simulink model "PowerLimiting_Saturation_LowPower"  (R2024a)
settings: Solver=VariableStepAuto  StartTime=0.0  StopTime=10  RelTol=1e-3
undefined symbols (not defined in the file or in its folder): Ion, Lithium
libraries: spsBatteryLib x1, spsControlledCurrentSourceLib x1, slpidlib x1, dspstat3 x1, spsVoltageMeasurementLib x1, simulink x1, sps_lib x1
settings Model: Creator=ezeki  LastModifiedBy=ezeki
settings DataIOCC: ExternalInput=[throttle]

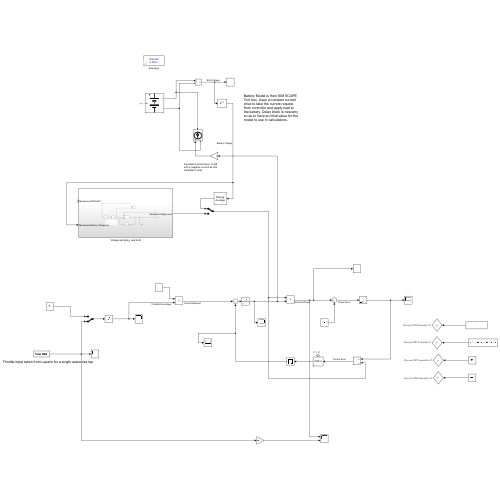
[thumbnail: Simulink's stored preview of the top-level diagram]
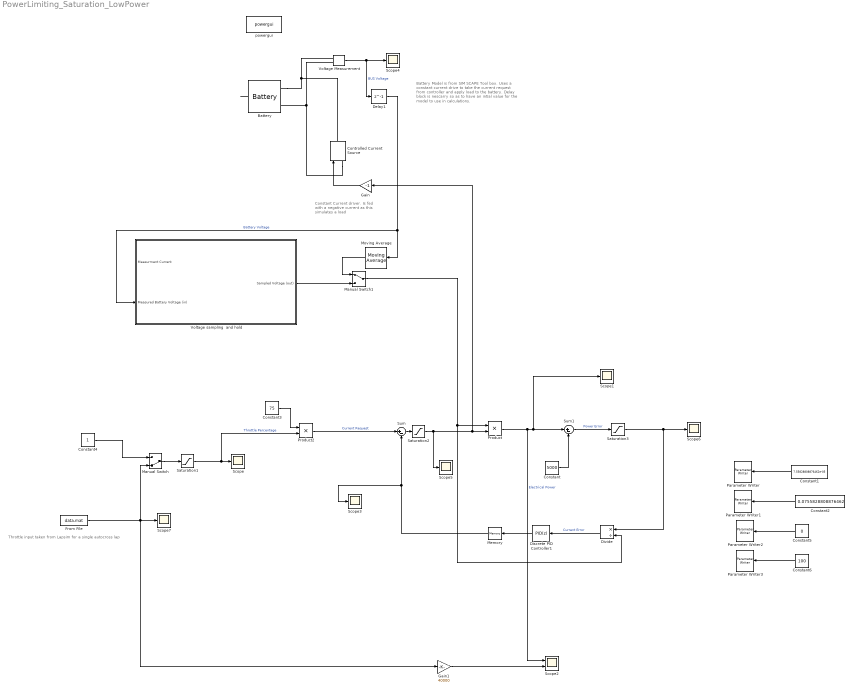
== system PowerLimiting_Saturation_LowPower ==
  note: Throttle input taken from Lapsim for a single autocross lap
  note: Constant Current driver. Is fed with a negative current as this simulates a load
  note: Battery Model is from SIM SCAPE Tool box. Uses a constant current drive to take the current request from controller and apply load to the battery. Delay block is nescarry so as to have an intial value for the model to use in calculations.
  Battery : spsBatteryLib/Battery  BatType=Lithium-Ion  ShowTempParam=off  ThermalPreset=no  ShowAgeParam=off  NomV=532.8  NomQ=1152  SOC=98.5  Batt_Tr=5  PresetModel=on  MaxQ=1152  MinV=399.6  FullV=620.1723  Dis_rate=500.8696  R=0.004625  Normal_OP=1041.8087  expZone="[575.6296      56.59826]"  current=[6.5 13 32.5]  Units=Time  Tci=20  NomT=20  T2=-30  MaxQ2=4.8  FullV2=7.1  Normal_OP2=5.655  expZone2="[6.58           1]"  Rca=0.6  ti=2000  Dp=0  Neq0=0  Tsim=1e6  Ta1=25  Qeol=5.4*0.9  Reol=0.013333*1.2  Char_age=[2.3478, 3]  Dis_age=[2.3478, 10]  N1=1500  N2=10500  N3=1000  N4=1400  Ta2=45  N5=950
  Constant : Constant  Value=5000
  Constant1 : Constant  Value=7.55828808876462e-05
  Constant2 : Constant  Value=0.0755828808876462
  Constant3 : Constant  Value=75
  Constant4 : Constant
  Constant5 : Constant  Value=0
  Constant6 : Constant  Value=100
  Controlled Current Source : spsControlledCurrentSourceLib/Controlled Current Source  Initialize=on  Source_Type=AC  Amplitude=0  Phase=0  Frequency=0  Measurements=None
  Delay1 : Delay  DelayLength=1  InitialCondition=600
  Discrete PID Controller1 : slpidlib/PID Controller  Controller=PID  Form=Parallel  TimeDomain=Discrete-time  UseExternalTs=off  SampleTime=-1  IntegratorMethod=Forward Euler  FilterMethod=Forward Euler  ControllerParametersSource=internal  P=1  I=1  UseKiTs=on  D=0  UseExternalDerivativeSource=off  N=100  UseFilter=on  TunerSelectOption=Transfer Function Based (PID Tuner App)  InitialConditionSource=internal  InitialConditionForIntegrator=60  InitialConditionForFilter=0  DifferentiatorICPrevScaledInput=0  ExternalReset=none  TrackingMode=off  Kt=1  LimitOutput=off  SatLimitsSource=internal  UpperSaturationLimit=inf  LowerSaturationLimit=-inf  LinearizeAsGain=off  AntiWindupMode=none  Kb=1  LimitIntegrator=off  UpperIntegratorSaturationLimit=inf  LowerIntegratorSaturationLimit=-inf  POutMin=[]  POutMax=[]  IOutMin=[]  IOutMax=[]  DOutMin=[]  DOutMax=[]  NOutMin=[]  NOutMax=[]  SumOutMin=[]  SumOutMax=[]  SaturationOutMin=[]  SaturationOutMax=[]  PParamMin=[]  PParamMax=[]  IParamMin=[]  IParamMax=[]  DParamMin=[]  DParamMax=[]  NParamMin=[]  NParamMax=[]  KbParamMin=[]  KbParamMax=[]  KtParamMin=[]  KtParamMax=[]  KbOutMin=[]  KbOutMax=[]  KtOutMin=[]  KtOutMax=[]  IntegratorOutMin=[]  IntegratorOutMax=[]  FilterOutMin=[]  FilterOutMax=[]  SumI1OutMin=[]  SumI1OutMax=[]  SumI2OutMin=[]  SumI2OutMax=[]  SumI3OutMin=[]  SumI3OutMax=[]  SumI4OutMin=[]  SumI4OutMax=[]  SumDOutMin=[]  SumDOutMax=[]  DifferentiatorOutMin=[]  DifferentiatorOutMax=[]  FilterDiffOutCoefMin=[]  FilterDiffOutCoefMax=[]  ReciprocalOutMin=[]  ReciprocalOutMax=[]  SumDenOutMin=[]  SumDenOutMax=[]  SumNumOutMin=[]  SumNumOutMax=[]  DivideOutMin=[]  DivideOutMax=[]  UdiffTsProdOutMin=[]  UdiffTsProdOutMax=[]  NTsProdOutMin=[]  NTsProdOutMax=[]  UintegralTsProdOutMin=[]  UintegralTsProdOutMax=[]  UngainTsProdOutMin=[]  UngainTsProdOutMax=[]  ClampingZeroOutDataTypeStr=Inherit: Inherit via back propagation  ClampingZeroOutMin=[]  ClampingZeroOutMax=[]  FilterDenConstantOutDataTypeStr=Inherit: Inherit via back propagation  FilterDenConstantOutMin=[]  FilterDenConstantOutMax=[]  PCopyOutDataTypeStr=Inherit: Inherit via back propagation  PCopyOutMin=[]  PCopyOutMax=[]  NCopyOutDataTypeStr=Inherit: Inherit via back propagation  NCopyOutMin=[]  NCopyOutMax=[]  IntegratorContinuousStateAttributes=''  IntegratorStateMustResolveToSignalObject=off  IntegratorRTWStateStorageClass=Auto  FilterContinuousStateAttributes=''  FilterStateMustResolveToSignalObject=off  FilterRTWStateStorageClass=Auto  ParallelPVariant=InternalParameters  IdealPVariant=Disabled  IVariant=InternalParameters  DVariant=InternalParameters  IntegratorVariant=Discrete  SatVariant=Disabled  AWVariant=Passthrough  PCopyVariant=Disabled  TRVariant=Disabled  FdbkBlocksVariant=Forward  IdealPFdbkVariant=Disabled  SatFdbkVariant=Disabled  DerivativeFilterVariant=ForwardEulerFilter  NVariant=InternalParameters  NCopyVariant=Disabled  FilterICVariant=InternalICsFilter  IntegratorICVariant=InternalICs  ExternalResetVariant=Disabled  TRSumVariant=Passthrough  SumFdbkVariant=Disabled  SumVariant=Sum_PID  TsampFilterVariant=InternalTs  TsampNgainVariant=Passthrough  TsampIntegralVariant=Disabled_SignalSpec  ExternalSaturationOutDataTypeStr=Inherit: Same as second input  DerivativeSourceVariant=ErrorSignal
      settings: LibrarySourceBlock=simulink/Discrete/Discrete PID Controller
  Divide : Product  Inputs=*/
  From File : FromFile  FileName=data.mat  SampleTime=0
  Gain : Gain  Gain=-1
  Gain1 : Gain  Gain=40000
  Manual Switch : ManualSwitch  CurrentSetting=0
  Manual Switch1 : ManualSwitch
  Memory : Memory  InitialCondition=14
  Moving Average : dspstat3/Moving Average  Method=Sliding window  ForgettingFactorPort=off  SpecifyWindowLength=on  WindowLength=10  OverlapLength=9  AllowArbitraryInputLength=off  ForgettingFactor=0.9  SimulateUsing=Interpreted execution
  Parameter Writer : ParameterWriter  ParameterOwnerBlock=../Discrete PID Controller1  ParameterName=P  ParameterInternalName=P
  Parameter Writer1 : ParameterWriter  ParameterOwnerBlock=../Discrete PID Controller1  ParameterName=I  ParameterInternalName=I
  Parameter Writer2 : ParameterWriter  ParameterOwnerBlock=../Discrete PID Controller1  ParameterName=D  ParameterInternalName=D
  Parameter Writer3 : ParameterWriter  ParameterOwnerBlock=../Discrete PID Controller1  ParameterName=N  ParameterInternalName=N
  Product : Product
  Product2 : Product
  Saturation1 : Saturate  UpperLimit=inf  LowerLimit=0
  Saturation2 : Saturate  UpperLimit=inf  LowerLimit=0
  Saturation3 : Saturate  UpperLimit=inf  LowerLimit=0
  Scope{,1,3..7} (7 alike) : Scope
  Scope2 : Scope  NumInputPorts=2
  Sum : Sum  Inputs=|+-
  Sum1 : Sum  Inputs=|+-
  Voltage Measurement : spsVoltageMeasurementLib/Voltage Measurement  PhasorSimulation=off  OutputType=Complex  PSBequivalent=0
  Voltage sampling  and hold : Subsystem
  powergui : sps_lib/powergui  Priority=1  SimulationMode=Discrete  SampleTime=0.002  frequency=60  Iterations=50  frequencyindice=0  Pbase=100e6  ErrMax=1e-4  UnitsV=kV  UnitsW=MW  buscounter=0  FunctionMessages=off  echomessages=off  EnableUseOfTLC=off  CurrentSourceSwitches=off  DisableSnubberDevices=off  DisableRonSwitches=off  DisableVfSwitches=off  DisplayEquations=off  AutomaticDiscreteSolvers=off  SolverType=Tustin/Backward Euler (TBE)  Interpol=off  ExternalGateDelay=off  methode=off  Ts=100  x0status=blocks  SPID=on  SwTol=0  HookPort=off  NonlinearTolerance=1e-4  nMaxIteration=100  ContinueOnMaxIteration=off  RestoreLinks=warning  ResistiveCurrentMeasurement=off  Frange=[0:2:500]  Ylog=off  Xlog=on  ShowGrid=off  save=off  variable=ZData  structure=0  ZoomFFT=off  StartTime=0.0  cycles=1  DisplayStyle=1  fundamental=60  FreqAxis=off  MaxFrequency=1000  frequencyindicesteady=1  RmsSteady=1  display=off
  wires:
  Saturation1/1 -> Scope/1, Product2/2  "Throttle Percentage"
  Constant4/1 -> Manual Switch/1
  Manual Switch/1 -> Saturation1/1
  Constant3/1 -> Product2/1
  Gain/1 -> Controlled Current Source/1
  Voltage Measurement/1 -> Delay1/1, Scope4/1  "BUS Voltage"
  Delay1/1 -> Voltage sampling  and hold/2(Measured Battery Voltage (in)), Moving Average/1  "Battery Voltage"
  Battery/1 -> ?
  From File/1 -> Manual Switch/2, Gain1/1, Scope7/1
  Product2/1 -> Sum/1  "Current Request"
  Voltage sampling  and hold/1(Sampled Voltage (out)) -> Manual Switch1/2
  Manual Switch1/1 -> Divide/2, Product/1
  Product/1 -> Scope1/1, Sum1/1, Scope2/1  "Electrical Power"
  Constant/1 -> Sum1/2
  Sum1/1 -> Saturation3/1  "Power Error"
  Divide/1 -> Discrete PID Controller1/1  "Current Error"
  Discrete PID Controller1/1 -> Memory/1
  Saturation2/1 -> Scope5/1, Gain/1, Product/2
  Moving Average/1 -> Manual Switch1/1
  Gain1/1 -> Scope2/2
  Memory/1 -> Scope3/1, Sum/2
  Sum/1 -> Saturation2/1
  Saturation3/1 -> Scope6/1, Divide/1
  Constant1/1 -> Parameter Writer/1
  Constant2/1 -> Parameter Writer1/1
  Constant5/1 -> Parameter Writer2/1
  Constant6/1 -> Parameter Writer3/1
  connections:
  Battery/LConn1 -- Voltage Measurement/LConn1 -- Controlled Current Source/RConn1
  Controlled Current Source/LConn1 -- Battery/LConn2 -- Voltage Measurement/LConn2

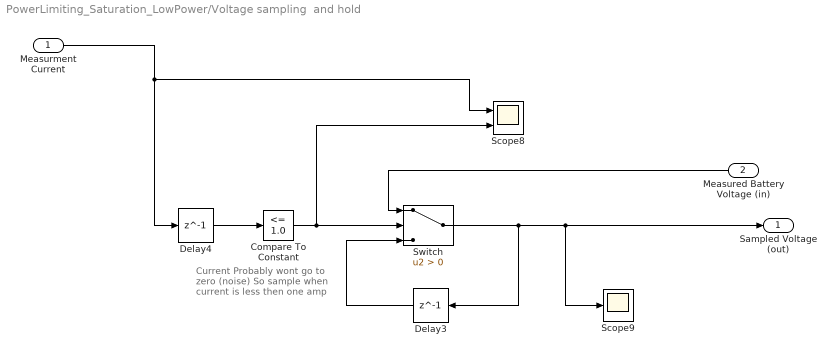
== system PowerLimiting_Saturation_LowPower/Voltage sampling  and hold ==
  note: Current Probably wont go to zero (noise) So sample when current is less then one amp
  Measurment Current : Inport
  Measured Battery Voltage (in) : Inport  Port=2
  Compare To Constant : simulink/Logic and Bit Operations/Compare To Constant  relop=<=  const=1.0  OutDataTypeStr=boolean
  Delay3 : Delay  DelayLength=1  InitialCondition=500
  Delay4 : Delay  DelayLength=1  InitialCondition=0
  Scope8 : Scope  NumInputPorts=2
  Scope9 : Scope
  Switch : Switch  Criteria=u2 > Threshold  SaturateOnIntegerOverflow=off  InputSameDT=off
  Sampled Voltage (out) : Outport
  wires:
  Compare To Constant/1 -> Scope8/2, Switch/2
  Measurment Current/1 -> Scope8/1, Delay4/1
  Delay3/1 -> Switch/3
  Switch/1 -> Delay3/1, Sampled Voltage (out)/1, Scope9/1
  Measured Battery Voltage (in)/1 -> Switch/1
  Delay4/1 -> Compare To Constant/1
